simulink model "specialBlocks"  (R2017b)
settings: Solver=FixedStepDiscrete  StartTime=0.0  StopTime=10.0  FixedStep=1  RelTol=1e-3
libraries: simulink x2
settings Model: Creator=cyarp  LastModifiedBy=cyarp

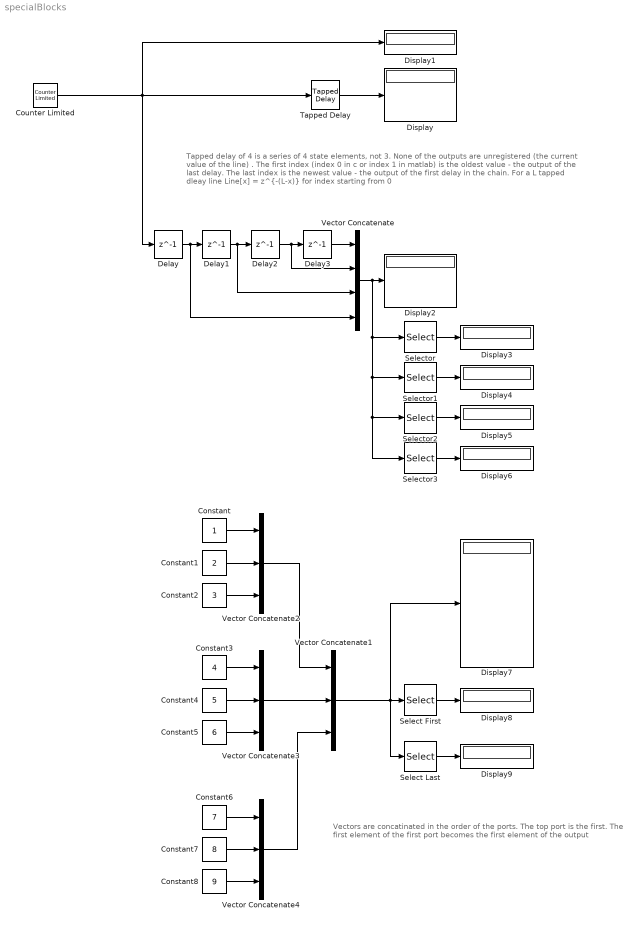
== system specialBlocks ==
  note: Vectors are concatinated in the order of the ports.  The top port is the first.
      | The first element of the first port becomes the first element of the output
  note: Tapped delay of 4 is a series of 4 state elements, not 3.  None of the outputs are unregistered (the current value of the line) .
      |
      | The first index (index 0 in c or index 1 in matlab) is the oldest value - the output of the last delay.
      | The last index is the newest value - the output of the first delay in the chain.
      |
      | For a L tapped dleay line
      | Line[x] = z^{-(L-x)} for index starting from 0
  Constant : Constant
  Constant1 : Constant  Value=2
  Constant2 : Constant  Value=3
  Constant3 : Constant  Value=4
  Constant4 : Constant  Value=5
  Constant5 : Constant  Value=6
  Constant6 : Constant  Value=7
  Constant7 : Constant  Value=8
  Constant8 : Constant  Value=9
  Counter Limited : simulink/Sources/Counter Limited  uplimit=31  tsamp=-1
  Delay{,1..3} (4 alike) : Delay  DelayLength=1
  Display{,1..9} (10 alike) : Display
  Select First : Selector  InputPortWidth=9  IndexOptions=Index vector (dialog)  Indices=[1]  OutputSizes=1
  Select Last : Selector  InputPortWidth=9  IndexOptions=Index vector (dialog)  Indices=[9]  OutputSizes=1
  Selector : Selector  InputPortWidth=4  IndexOptions=Index vector (dialog)  Indices=[1]  OutputSizes=1
  Selector1 : Selector  InputPortWidth=4  IndexOptions=Index vector (dialog)  Indices=[2]  OutputSizes=1
  Selector2 : Selector  InputPortWidth=4  IndexOptions=Index vector (dialog)  Indices=[3]  OutputSizes=1
  Selector3 : Selector  InputPortWidth=4  IndexOptions=Index vector (dialog)  Indices=[4]  OutputSizes=1
  Tapped Delay : simulink/Discrete/Tapped Delay  vinit=0.0  samptime=-1  NumDelays=4  DelayOrder=Oldest  includeCurrent=off
  Vector Concatenate : Concatenate  NumInputs=4
  Vector Concatenate{1..4} (4 alike) : Concatenate  NumInputs=3
  wires:
  Counter Limited/1 -> Tapped Delay/1, Display1/1, Delay/1
  Tapped Delay/1 -> Display/1
  Delay/1 -> Vector Concatenate/4, Delay1/1
  Delay1/1 -> Vector Concatenate/3, Delay2/1
  Delay2/1 -> Vector Concatenate/2, Delay3/1
  Vector Concatenate/1 -> Selector2/1, Selector3/1, Selector1/1, Selector/1, Display2/1
  Delay3/1 -> Vector Concatenate/1
  Selector/1 -> Display3/1
  Selector1/1 -> Display4/1
  Selector2/1 -> Display5/1
  Selector3/1 -> Display6/1
  Constant/1 -> Vector Concatenate2/1
  Constant1/1 -> Vector Concatenate2/2
  Constant2/1 -> Vector Concatenate2/3
  Vector Concatenate2/1 -> Vector Concatenate1/1
  Constant3/1 -> Vector Concatenate3/1
  Constant4/1 -> Vector Concatenate3/2
  Constant5/1 -> Vector Concatenate3/3
  Vector Concatenate3/1 -> Vector Concatenate1/2
  Vector Concatenate4/1 -> Vector Concatenate1/3
  Constant6/1 -> Vector Concatenate4/1
  Constant7/1 -> Vector Concatenate4/2
  Constant8/1 -> Vector Concatenate4/3
  Vector Concatenate1/1 -> Select Last/1, Select First/1, Display7/1
  Select First/1 -> Display8/1
  Select Last/1 -> Display9/1
